simulink library "casper_library_correlator"  (Simulink 7.0)
libraries: xbsIndex_r4 x1223, xbsReplacements_r4 x72, casper_library_misc x59, casper_library_multipliers x32, xps_library x8, casper_library_correlator x3, casper_library_delays x2
(part 1 of 12)
settings Model: Creator=mdexter  LastModifiedBy=mdexter

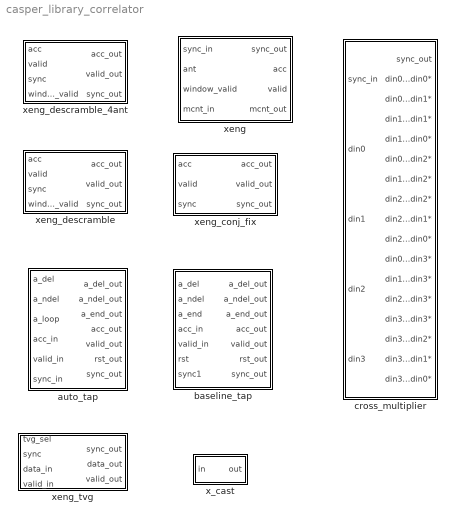
== system casper_library_correlator ==
  auto_tap : Subsystem  mask(auto_tap){n_ants=4, n_bits=4, acc_len=32, add_latency=1, mult_latency=2, bram_latency=2, use_ded_mult=1, use_bram_delay=1}
      mask prompts: n_ants "Number of antennas"; n_bits "Number of input bits (per complex component)"; acc_len "Accumulation length"; add_latency "Adder latency"; mult_latency "Multiplier latency"; bram_latency "BRAM latency"; use_ded_mult "Use Dedicated Multipliers"; use_bram_delay "Implementation: Delay type (0=SLR, 1=BRAM)"
      mask init:
      | fix_pnt_pos = (n_bits-1)*2;
      | bit_growth = ceil(log2(acc_len));
      | ant_bits = ceil(log2(n_ants));
      | n_bits_out = (2*n_bits + 1 + bit_growth);
      | 
      | 
      | auto_tap_init(gcb, ...
      |     'use_ded_mult', use_ded_mult, ...
      |     'use_bram_delay', use_bram_delay);
      settings: AttributesFormatString=mult=1
  baseline_tap : Subsystem  mask(baseline_tap){n_ants=4, ant_sep=1, n_bits=4, acc_len=32, add_latency=1, mult_latency=2, bram_latency=2, use_ded_mult=1, use_bram_delay=1}
      mask prompts: n_ants "Number of antennas"; ant_sep "Antenna Seperation"; n_bits "number of input bits (per complex component)"; acc_len "accumulation length"; add_latency "Adder latency"; mult_latency "Multiplier latency"; bram_latency "BRAM latency"; use_ded_mult "Multiplier Type (0=slices 1=embedded 2=bram)"; use_bram_delay "Use BRAM delays"
      mask init:
      | fix_pnt_pos = (n_bits-1)*2;
      | bit_growth = ceil(log2(acc_len));
      | ant_bits = ceil(log2(n_ants));
      | n_bits_out = (2*n_bits + 1 + bit_growth);
      | 
      | baseline_tap_init(gcb, ...
      |     'ant_sep', ant_sep, ...
      |     'use_ded_mult', use_ded_mult, ...
      |     'use_bram_delay', use_bram_delay);
      settings: AttributesFormatString=ant_sep=1, mult=1, bram=1
  cross_multiplier : Subsystem  mask(cross_multiplier){streams=4, aggregation=2, bit_width_in=4, binary_point_in=3, bit_width_out=9, binary_point_out=6, mult_latency=2, add_latency=1, overflow=Wrap, quantisation=Truncate, conv_latency=0}
      mask prompts: streams "Number input streams"; aggregation "Aggregation per stream"; bit_width_in "Bit width in"; binary_point_in "Binary point in"; bit_width_out "Bit width out"; binary_point_out "Binary point out"; mult_latency "Multiplier latency"; add_latency "Adder latency"; overflow "Overflow behaviour"; quantisation "Quantisation behaviour"; conv_latency "Bit width conversion latency"
      mask help: Cross multiplies aggregated complex input streams.
      mask init:
      | cross_multiplier_init(gcb, ...
      |     'streams', streams, ...
      |     'aggregation', aggregation, ...
      |     'bit_width_in', bit_width_in, ...
      |     'binary_point_in', binary_point_in, ...
      |     'bit_width_out', bit_width_out, ...
      |     'binary_point_out', binary_point_out, ...
      |     'mult_latency', mult_latency, ...
      |     'add_latency', add_latency, ...
      |     'overflow', overflow, ...
      |     'quantisation', quantisation, ...
      |     'conv_latency', conv_latency);
      mask StyleString: edit,edit,edit,edit,edit,edit,edit,edit,popup(Wrap|Saturate|Error),popup(Truncate|Round  (unbiased: +/- Inf)|Round  (unbiased: even values)),edit
  x_cast : Subsystem  mask{n_bits_in=16, n_bits_out=16, fix_pnt_pos=6, demux_factor=8}
      mask prompts: n_bits_in "Number of bits (input)"; n_bits_out "Number of bits (output)"; fix_pnt_pos "Fixed point position"; demux_factor "Demux Factor"
      mask init:
      | switch (demux_factor)
      |     case (8)
      |         bit_offsets=[0 1 2 3 4 5 6 7];
      |     case (4) 
      |         bit_offsets=[4 5 6 7 0 1 2 3];  
      |     case (2) 
      |         bit_offsets=[6 7 4 5 2 3 0 1];  
      |     case (1) 
      |         bit_offsets=[7 6 5 4 3 2 1 0];  
      | end
  xeng : Subsystem  mask(xeng){n_ants=4, n_bits=4, acc_len=32, demux_factor=1, add_latency=1, mult_latency=2, bram_latency=2, use_ded_mult=1, use_bram_delay=1}
      mask prompts: n_ants "Number of antennas"; n_bits "Bit-width of samples in"; acc_len "Accumulation length"; add_latency "Adder latency"; mult_latency "Multiplier latency"; bram_latency "BRAM latency"; use_ded_mult "Implementation: Multiplier type (0=slices 1=embedded 2=bram)"; use_bram_delay "Implementation: Delay type (0=SLR, 1=BRAM)"
      mask help: CASPER X engine with added internal valid data masking functionality, descramble and integral demux. Based on Aaron Parsons' and Lynn Urry's original X engine design.
      mask init:
      | xeng_init(gcb, ...
      |     'n_ants', n_ants, ...
      |     'n_bits', n_bits, ...
      |     'acc_len', acc_len, ...
      |     'demux_factor', demux_factor, ...
      |     'add_latency', add_latency, ...
      |     'mult_latency', mult_latency, ...
      |     'bram_latency', bram_latency, ...
      |     'use_ded_mult', use_ded_mult, ...
      |     'use_bram_delay', use_bram_delay);
      settings: AttributesFormatString=n_ant=4, bits=4, mult=1, bram=1
      mask StyleString: edit,edit,edit,popup(1|2|4|8),edit,edit,edit,edit,edit
  xeng_conj_fix : Subsystem  mask(xeng_conj_fix){n_ants=8, n_bits_in=4, demux_factor=8}
      mask prompts: n_ants "Number of Antennas"; n_bits_in "Input Bitwidth (complex, bit width per component)"; demux_factor "Demux factor"
      mask help:
      | This block corrects the "lower triangle" of the X engine's output so that products are conjugated according to the astronomy convention of
      | lower_antenna_index * conj(higher_antenna_index).
      |
      | It expects demuxed input. Ie the ACC line contains a single complex number per clock.
      mask init:
      | xeng_conj_fix_init(gcb, 'n_ants', n_ants,...
      |     'n_bits_in',n_bits_in,...
      |     'demux_factor',demux_factor);
      | 
      | fmtstr = sprintf('num_ants=%d',n_ants);
      | set_param(gcb, 'AttributesFormatString', fmtstr);
      settings: AttributesFormatString=num_ants=8
  xeng_descramble : Subsystem  mask(xeng_descramble){num_ants=8, n_bits_in=128, demux_factor=8, acc_len=128}
      mask prompts: num_ants "Number of Antennas"; n_bits_in "Input Bitwidth"; demux_factor "Demux factor"; acc_len "X engine accumulation length"
      mask help:
      | NOT TESTED FOR non-2^N antennas.
      |
      | Descrambles X engine output. Optionally demuxes output.
      mask init:
      | num_taps = floor(num_ants/2) + 1;
      | ant_bits = ceil(log2(num_ants));
      | num_validins = num_ants*num_taps;
      | validin_bits = floor(log2(num_validins))+1;
      | demux_bits = floor(log2(demux_factor))+1;
      | acc_len_bits = floor(log2(acc_len))+1;
      | num_ants_bits = floor(log2(num_ants))+1;
      | taps_bits = floor(log2(num_taps))+1;
      | pivot_pnt = num_ants/2*(num_taps) + num_taps*num_ants/4;
      | num_elements = nchoosek(num_ants, 2) + num_ants;
      | elements_bits = floor(log2(num_elements)) + 1;
      | 
      | ship_el_del = floor(acc_len*num_ants/num_validins/demux_factor) - 1;
      | 
      | if (ship_el_del < 0)
      |     errordlg('Insufficient output space for this configuration. Try a lower demux setting. Else you need fewer antennas or longer xeng acc time.');
      |     ship_el_del=0
      | end
      | 
      | if (ship_el_del == 0)
      |     ship_el_cnt = demux_factor*num_elements-1;
      |     %in this case we're outputting multiple words back-to-back.
      | else
      |     ship_el_cnt = demux_factor*num_elements;
      |     %in this case we're outputting one word at a time.
      | end
      | 
      | ship_el_del_bits = ceil(log2(ship_el_del + 1));
      | 
      | if (ship_el_del_bits == 0)
      |     ship_el_del_bits =1;
      | end
      | 
      | fmtstr = sprintf('num_ants=%d',num_ants);
      | set_param(gcb, 'AttributesFormatString', fmtstr);
      settings: AttributesFormatString=num_ants=8
  xeng_descramble_4ant : Subsystem  mask(xeng_descramble){n_bits_in=128, demux_factor=8, acc_len=32}
      mask prompts: n_bits_in "Input Bitwidth"; demux_factor "Demux factor"; acc_len "X engine accumulation length"
      mask help:
      | NOT TESTED FOR non-2^N antennas.
      |
      | Descrambles X engine output. Optionally demuxes output.
      mask init:
      | num_ants = 4;
      | num_taps = floor(num_ants/2) + 1;
      | ant_bits = ceil(log2(num_ants));
      | num_validins = num_ants*num_taps;
      | validin_bits = floor(log2(num_validins))+1;
      | demux_bits = floor(log2(demux_factor))+1;
      | acc_len_bits = floor(log2(acc_len))+1;
      | num_ants_bits = floor(log2(num_ants))+1;
      | taps_bits = floor(log2(num_taps))+1;
      | pivot_pnt = num_ants/2*(num_taps) + num_taps*num_ants/4;
      | num_elements = nchoosek(num_ants, 2) + num_ants;
      | elements_bits = floor(log2(num_elements)) + 1;
      | 
      | ship_el_del = floor(acc_len*num_ants/num_validins/demux_factor) - 1;
      | 
      | if (ship_el_del < 0)
      |     errordlg('Insufficient output space for this configuration. Try a lower demux setting. Else you need fewer antennas or longer xeng acc time.');
      |     ship_el_del=0
      | end
      | 
      | if (ship_el_del == 0)
      |     ship_el_cnt = demux_factor*num_elements-1;
      |     %in this case we're outputting multiple words back-to-back.
      | else
      |     ship_el_cnt = demux_factor*num_elements;
      |     %in this case we're outputting one word at a time.
      | end
      | 
      | ship_el_del_bits = ceil(log2(ship_el_del + 1));
      | 
      | if (ship_el_del_bits == 0)
      |     ship_el_del_bits =1;
      | end
      | 
      | fmtstr = sprintf('num_ants=%d',num_ants);
      | set_param(gcb, 'AttributesFormatString', fmtstr);
      settings: AttributesFormatString=num_ants=4
  xeng_tvg : Subsystem  mask{ant_bits=2, x_int_bits=5, sync_period=15}
      mask prompts: ant_bits "Number of Antennas (2^?):"; x_int_bits "X Integration Length (2^?):"; sync_period "Sync Pulse Period (2^?):"

== system casper_library_correlator/auto_tap ==
  a_del : Inport  OutDataType=sfix(16)  OutScaling=2^0
  a_ndel : Inport  Port=2  OutDataType=sfix(16)  OutScaling=2^0
  a_loop : Inport  Port=3  OutDataType=sfix(16)  OutScaling=2^0
  acc_in : Inport  Port=4  OutDataType=sfix(16)  OutScaling=2^0
  valid_in : Inport  Port=5  OutDataType=sfix(16)  OutScaling=2^0
  sync_in : Inport  Port=6  OutDataType=sfix(16)  OutScaling=2^0
  delay : Subsystem  AncestorBlock=casper_library_delays/delay_bram  mask(delay_bram){DelayLen=(acc_len - 1)*ceil(n_ants/2) + ceil(n_ants/2)-floor(n_ants/2), bram_latency=bram_latency, use_dsp48=off}
      mask prompts: DelayLen "Delay By:"; bram_latency "BRAM Latency"; use_dsp48 "Use DSP48"
      mask help: A delay block that uses BRAM for its storage.
      mask init:
      | if (DelayLen <= bram_latency)
      | 	error('delay value must be greater than BRAM Latency');
      | end
      | BitWidth = max(ceil(log2(DelayLen)), 2);
      | if strcmp(use_dsp48,'on'),
      |     set_param([gcb,'/Counter'], 'use_behavioral_HDL', 'off', ...
      |         'use_rpm', 'on', 'implementation', 'DSP48');
      | else, %default counter settings
      |         set_param([gcb,'/Counter'], 'use_behavioral_HDL', 'off', ...
      |         'use_rpm', 'off', 'implementation', 'Fabric');
      | end
      mask Help: eval('xlWeb(''http://casper.berkeley.edu/wiki/Delay_bram'')')
  dual_pol_cmac : Subsystem
  sync_delay : casper_library_delays/sync_delay  SystemSampleTime=-1  DelayLen=add_latency + mult_latency + acc_len + floor(n_ants/2 + 1) + 1
      link override Constant: equ=P=C
      link override Constant1: equ=P=C
      link override Constant2: equ=P=C
      link override Constant3: equ=P=C
  a_del_out : Outport  OutDataType=sfix(16)  OutScaling=2^0
  a_ndel_out : Outport  Port=2  OutDataType=sfix(16)  OutScaling=2^0
  a_end_out : Outport  Port=3  OutDataType=sfix(16)  OutScaling=2^0
  acc_out : Outport  Port=4  OutDataType=sfix(16)  OutScaling=2^0
  valid_out : Outport  Port=5  OutDataType=sfix(16)  OutScaling=2^0
  rst_out : Outport  Port=6  OutDataType=sfix(16)  OutScaling=2^0
  sync_out : Outport  Port=7  OutDataType=sfix(16)  OutScaling=2^0
  wires:
  sync_in/1 -> sync_delay/1, dual_pol_cmac/4(sync), rst_out/1
  a_del/1 -> dual_pol_cmac/1(a1), a_del_out/1
  dual_pol_cmac/1(acc_out) -> acc_out/1
  acc_in/1 -> dual_pol_cmac/3(acc_in)
  dual_pol_cmac/2(valid_out) -> valid_out/1
  valid_in/1 -> dual_pol_cmac/5(valid_in)
  a_ndel/1 -> dual_pol_cmac/2(a2), a_ndel_out/1
  a_loop/1 -> delay/1(In1)
  delay/1(Out1) -> a_end_out/1
  sync_delay/1 -> sync_out/1

== system casper_library_correlator/baseline_tap ==
  a_del : Inport  OutDataType=sfix(16)  OutScaling=2^0
  a_ndel : Inport  Port=2  OutDataType=sfix(16)  OutScaling=2^0
  a_end : Inport  Port=3  OutDataType=sfix(16)  OutScaling=2^0
  acc_in : Inport  Port=4  OutDataType=sfix(16)  OutScaling=2^0
  valid_in : Inport  Port=5  OutDataType=sfix(16)  OutScaling=2^0
  rst : Inport  Port=6  OutDataType=sfix(16)  OutScaling=2^0
  sync1 : Inport  Port=7  OutDataType=sfix(16)  OutScaling=2^0
  Constant : xbsIndex_r4/Constant  arith_type=Unsigned  const=ant_sep * acc_len  n_bits=ant_bits + bit_growth  bin_pt=0  explicit_period=off  period=1  equ=P=C  opselect=C  inp2=PCIN>>17  opr=+  inp1=P  carry=CIN  dbl_ovrd=off  block_type=constant
      settings: block_version=9.1.01
  Convert : xbsIndex_r4/Convert  arith_type=Unsigned  n_bits=1  bin_pt=0  quantization=Truncate  overflow=Wrap  latency=0  dbl_ovrd=off  pipeline=off  block_type=convert
      settings: xl_area=[0, 0, 0, 0, 0, 0, 0]
  Counter : xbsIndex_r4/Counter  cnt_type=Count Limited  cnt_to=n_ants * acc_len - 1  operation=Up  start_count=0  cnt_by_val=1  arith_type=Unsigned  n_bits=ant_bits + bit_growth  bin_pt=0  load_pin=off  rst=on  en=off  explicit_period=off  period=1  dbl_ovrd=off  use_behavioral_HDL=off  implementation=Fabric  use_rpm=on  block_type=counter
      settings: xl_area=[0, 0, 0, 0, 0, 0, 0]  block_version=9.1.01
  Delay{1,3,7..8} (4 alike) : xbsIndex_r4/Delay  en=off  latency=1  dbl_ovrd=off  reg_retiming=on  block_type=delay
      settings: xl_area=[0, 0, 0, 0, 0, 0, 0]  block_version=9.1.01
  Mux : xbsIndex_r4/Mux  inputs=2  en=off  latency=1  precision=Full  arith_type="Signed  (2's comp)"  n_bits=8  bin_pt=2  quantization=Truncate  overflow=Wrap  dbl_ovrd=off  block_type=mux
      settings: xl_area=[0, 0, 0, 0, 0, 0, 0]  block_version=9.1.01
  Relational : xbsIndex_r4/Relational  mode=a<b  en=off  latency=0  dbl_ovrd=off  block_type=relational
      settings: xl_area=[0, 0, 0, 0, 0, 0, 0]  block_version=9.1.01
  delay : Subsystem  AncestorBlock=casper_library_delays/delay_bram  mask(delay_bram){DelayLen=acc_len, bram_latency=bram_latency, use_dsp48=off}
      mask prompts: DelayLen "Delay By:"; bram_latency "BRAM Latency"; use_dsp48 "Use DSP48"
      mask help: A delay block that uses BRAM for its storage.
      mask init: same as casper_library_correlator/auto_tap/delay
      mask Help: eval('xlWeb(''http://casper.berkeley.edu/wiki/Delay_bram'')')
  dual_pol_cmac : Subsystem
  a_del_out : Outport  OutDataType=sfix(16)  OutScaling=2^0
  a_ndel_out : Outport  Port=2  OutDataType=sfix(16)  OutScaling=2^0
  a_end_out : Outport  Port=3  OutDataType=sfix(16)  OutScaling=2^0
  acc_out : Outport  Port=4  OutDataType=sfix(16)  OutScaling=2^0
  valid_out : Outport  Port=5  OutDataType=sfix(16)  OutScaling=2^0
  rst_out : Outport  Port=6  OutDataType=sfix(16)  OutScaling=2^0
  sync_out : Outport  Port=7  OutDataType=sfix(16)  OutScaling=2^0
  wires:
  sync1/1 -> sync_out/1
  Delay1/1 -> rst_out/1, dual_pol_cmac/4(sync)
  Delay8/1 -> a_end_out/1
  Delay7/1 -> a_ndel_out/1
  Delay3/1 -> a_del_out/1, dual_pol_cmac/1(a1)
  a_end/1 -> Delay8/1, Mux/3
  a_ndel/1 -> Delay7/1, Mux/2
  valid_in/1 -> dual_pol_cmac/5(valid_in)
  dual_pol_cmac/2(valid_out) -> valid_out/1
  acc_in/1 -> dual_pol_cmac/3(acc_in)
  dual_pol_cmac/1(acc_out) -> acc_out/1
  a_del/1 -> delay/1(In1)
  rst/1 -> Counter/1, Delay1/1
  Convert/1 -> Mux/1
  Relational/1 -> Convert/1
  Constant/1 -> Relational/2
  Counter/1 -> Relational/1
  Mux/1 -> dual_pol_cmac/2(a2)
  delay/1(Out1) -> Delay3/1
